simulink library "gmp_sil_core_pack_src"  (R2022b)
settings: Solver=VariableStepAuto  StartTime=0.0  StopTime=10.0  RelTol=1e-3
libraries: sm_lib x5, nesl_utility x4, fl_lib x3, peripheral_utilities x1, gmp_sil_core_pack x1
settings Model: Creator=javnson  LastModifiedBy=javnson

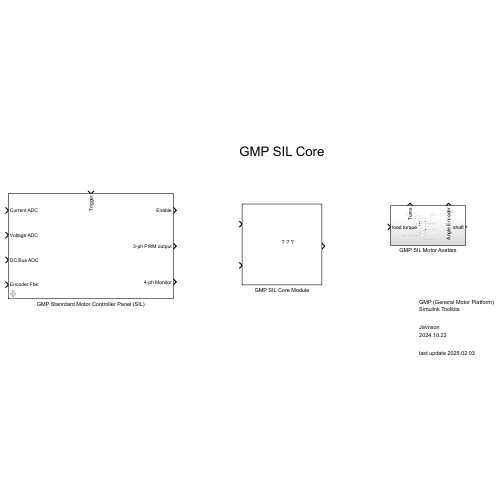
[thumbnail: Simulink's stored preview of the top-level diagram]
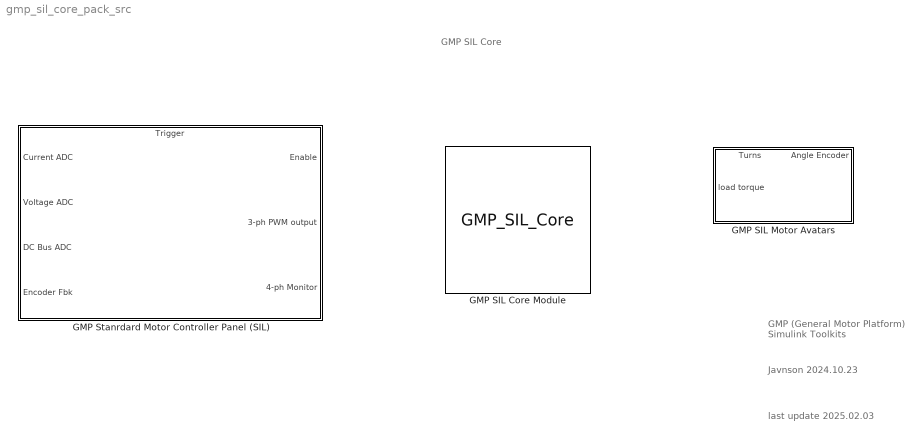
== system gmp_sil_core_pack_src ==
  note: last update 2025.02.03
  note: GMP SIL Core
  note: Javnson
      | 2024.10.23
  note: GMP (General Motor Platform)
      | Simulink Toolkits
  GMP SIL Core Module : S-Function  FunctionName=GMP_SIL_Core  Parameters=NumberUnpackedPorts, UnpackedDataTypes, UnpackedDataSizes, NumberPackedPorts, PackedDataTypes, PackedDataSizes, Alignment, HostAddr, TargetPort  SFunctionDeploymentMode=off  EnableBusSupport=off  mask(GMP CTL SIL Core){MaskPackedDataTypes={'double','double'}, MaskPackedDataSizes={[1],[1]}, MaskUnpackedDataTypes={'double'}, MaskUnpackedDataSizes={[1]}, MaskAlignment=1, MaskHostAddr='127.0.0.1', MaskMsgTxPort=12300, MaskMsgRxPort=12301, MaskCmdTxPort=12302, MaskCmdRxPort=12303}
      mask help:
      | This is the GMP (General Motor Platform) CTL (Control Template Library) SIL (Software In Loop) Core Model.
      | User should fill the following communication settings.
      mask init:
      | % MDL invoke parameters
      | % NumberUnpackedPorts, UnpackedDataTypes, UnpackedDataSizes, 
      | % NumberPackedPorts, PackedDataTypes, PackedDataSizes, 
      | % Alignment,
      | % HostAddr, TargetPort
      | 
      | % source: MaskUnpackedDataTypes, MaskUnpackedDataSizes
      | % source: MaskPackedDataTypes, MaskUnpackedDataSizes
      | % source: MaskAlignment
      | [NumberUnpackedPorts, UnpackedDataTypes, UnpackedDataSizes, ...
      |      NumberPackedPorts, PackedDataTypes, PackedDataSizes, ...
      |      Alignment] = mdl_gmp_simulink_core( ...
      |      MaskUnpackedDataTypes, MaskUnpackedDataSizes, ...
      |      MaskPackedDataTypes, MaskPackedDataSizes,...
      |      MaskAlignment);
      | 
      | % source: MaskHostAddr
      | % source: MaskMsgTxPort, MaskMsgRxPort
      | % source: MaskCmdTxPort, MaskCmdRxPort
      | [HostAddr, TargetPort] = mdl_gmp_simulink_connection(MaskHostAddr, ...
      | 	MaskMsgTxPort, MaskMsgRxPort, ... 
      | 	MaskCmdTxPort, MaskCmdRxPort);
      mask TypeOptions MaskAlignment: 1 | 2 | 4 | 8
      mask DialogControl ParameterGroupVar Prompt: Parameters:
      mask DialogControl Container5 Prompt: Message
      mask DialogControl Control3 Prompt: Data (sent) types (cell array):(pack)
      mask DialogControl Control7 Prompt: Data (send) port dimisions (cell array) (pack), disabled
      mask DialogControl Control5 Prompt: Data (received) types (cell array):(unpack)
      mask DialogControl Control6 Prompt: Data (received) port dimisions (cell array)(unpacked)
      mask DialogControl Control4 Prompt: Byte Alignment:
      mask DialogControl Container6 Prompt: Connection
      mask DialogControl Control8 Prompt: Target Host:
      mask DialogControl Control9 Prompt: MSG Transmit Port:
      mask DialogControl Control10 Prompt: MSG Receive Port:
      mask DialogControl Container7 Prompt: Command Ports
      mask DialogControl Control11 Prompt: CMD Transmit Port:
      mask DialogControl Control12 Prompt: CMD Receive Port:
      mask Display:
      | image(append(fileparts(which('gmp_simulink_utilities.slx')),'\icon\GMP_Core.png'));
      | 
      | 
      | disp('\n\n\n\n\n\n\n\nGMP SIL CORE Module');
  GMP SIL Motor Avatars : Subsystem
      settings: PortSchema="{\"entries\":[{\"content\":{\"sides\":[{\"content\":{\"connectorIds\":[\"In1\"]},\"type\":\"ConnectorPlacement.EquallySpacedRectSide\",\"uuid\":\"93fd98c8-22a3-43d8-9c64-5fedb21a7bba\"},{\"content\":{\"connectorIds\":[\"RConn1\"],\"side\":\"RIGHT\"},\"type\":\"ConnectorPlacement.EquallySpacedRectSide\",\"uuid\":\"d117f16d-9ccc-4fe6-b623-9fd4cd524b7a\"},{\"content\":{\"connectorIds\":[\"Out1\",\"Out2\"],\"side\":\"TOP\"},\"type\":\"ConnectorPlacement.EquallySpacedRectSide\",\"uuid\":\"de5de415-7a5e-456c-8b58-b022e0bdb100\"}]},\"type\":\"ConnectorPlacement.EquallySpacedConnector\",\"uuid\":\"15174bc1-c3ff-4fbf-b424-15a1ef65b97f\"}],\"packageUris\":[\"http://schema.mathworks.com/mf0/Connector/R2020b\"],\"version\":\"1.0\"}"
  GMP Stanrdard Motor Controller Panel (SIL) : Subsystem  mask(GMP SIL Core for single Motor Controller){}
      mask help: This is a General GMP SIL Motor Simulator.
      settings: PortSchema="{\"entries\":[{\"content\":{\"sides\":[{\"content\":{\"connectorIds\":[\"In1\",\"In2\",\"In3\",\"In4\"]},\"type\":\"ConnectorPlacement.EquallySpacedRectSide\",\"uuid\":\"92070e77-c4d8-4bd6-a20f-015d90d53703\"},{\"content\":{\"connectorIds\":[\"Out1\",\"Out2\",\"Out3\"],\"side\":\"RIGHT\"},\"type\":\"ConnectorPlacement.EquallySpacedRectSide\",\"uuid\":\"cd227558-01ea-4976-b12d-cc815f5c8239\"},{\"content\":{\"connectorIds\":[\"In5\"],\"side\":\"TOP\"},\"type\":\"ConnectorPlacement.EquallySpacedRectSide\",\"uuid\":\"6d86fdab-8964-4d81-bb99-d1a603f01c68\"}]},\"type\":\"ConnectorPlacement.EquallySpacedConnector\",\"uuid\":\"4dd76185-b108-46e1-8d6d-0c6e9edd0ad4\"}],\"packageUris\":[\"http://schema.mathworks.com/mf0/Connector/R2020b\"],\"version\":\"1.0\"}"

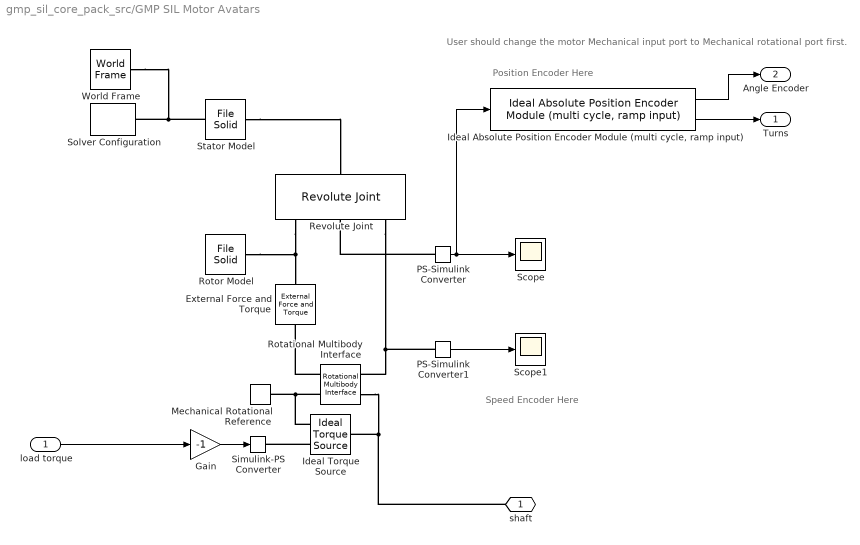
== system gmp_sil_core_pack_src/GMP SIL Motor Avatars ==
  note: User should change the motor Mechanical input port to Mechanical rotational port first.
  note: Speed Encoder Here
  note: Position Encoder Here
  load torque : Inport
  External Force and Torque : sm_lib/Forces and Torques/External Force and Torque  EnableForceX=off  EnableForceY=off  EnableForceZ=off  EnableForce=off  ForceResolutionFrame=AttachedFrame  EnableTorqueX=off  EnableTorqueY=off  EnableTorqueZ=on  EnableTorque=off  TorqueResolutionFrame=AttachedFrame
  Gain : Gain  Gain=-1
  "Ideal Absolute Position Encoder Module (multi cycle, ramp input)" : peripheral_utilities/Ideal Absolute Position Encoder Module (multi cycle, ramp input)  ENCODER_BIT=17
  Ideal Torque Source : fl_lib/Mechanical/Mechanical Sources/Ideal Torque Source
  Mechanical Rotational Reference : fl_lib/Mechanical/Rotational Elements/Mechanical Rotational Reference
  PS-Simulink Converter : nesl_utility/PS-Simulink Converter  PhysicalDomain=network_engine_domain  SubClassName=ps_output  LeftPortType=input  RightPortType=output  PseudoPeriodic=off  Frequencies=[]  VectorFormat=inherit  Unit=inherit  AffineConversion=off
  PS-Simulink Converter1 : nesl_utility/PS-Simulink Converter  PhysicalDomain=network_engine_domain  SubClassName=ps_output  LeftPortType=input  RightPortType=output  PseudoPeriodic=off  Frequencies=[]  VectorFormat=inherit  Unit=inherit  AffineConversion=off
  Revolute Joint : sm_lib/Joints/Revolute Joint  JointMode=Normal  CompositeWrenchDir=FollowerOnBase  CompositeWrenchFrame=BaseFrame  SenseConstraintForce=off  SenseConstraintTorque=off  SenseTotalForce=off  SenseTotalTorque=off  PositionTargetSpecify=off  PositionTargetPriority=High  PositionTargetValue=0  PositionTargetValueUnits=deg  VelocityTargetSpecify=off  VelocityTargetPriority=High  VelocityTargetValue=0  VelocityTargetValueUnits=deg/s  EquilibriumPosition=0  EquilibriumPositionUnits=deg  SpringStiffness=0  SpringStiffnessUnits=N*m/deg  DampingCoefficient=0  DampingCoefficientUnits=N*m/(deg/s)  LowerLimitSpecify=off  LowerLimitBound=-90  LowerLimitBoundUnits=deg  LowerLimitStiffness=1e4  LowerLimitStiffnessUnits=N*m/deg  LowerLimitDamping=10  LowerLimitDampingUnits=N*m/(deg/s)  LowerLimitTransitionRegionWidth=0.1  LowerLimitTransitionRegionWidthUnits=deg  UpperLimitSpecify=off  UpperLimitBound=90  UpperLimitBoundUnits=deg  UpperLimitStiffness=1e4  UpperLimitStiffnessUnits=N*m/deg  UpperLimitDamping=10  UpperLimitDampingUnits=N*m/(deg/s)  UpperLimitTransitionRegionWidth=0.1  UpperLimitTransitionRegionWidthUnits=deg  TorqueActuationMode=NoTorque  MotionActuationMode=ComputedMotion  SensePosition=on  SenseVelocity=on  SenseAcceleration=off  SenseTorqueForce=off  SenseLowerLimitTorqueForce=off  SenseUpperLimitTorqueForce=off
  Rotational Multibody Interface : fl_lib/Mechanical/Multibody Interfaces/Rotational Multibody Interface
  Rotor Model : sm_lib/Body Elements/File Solid  ExtGeomFileName=resources\rotor.STEP  UnitType=FromFile  ExtGeomFileUnits=m  StepReaderType=HEX  ExportConvexHullGeometry=off  InertiaType=CalculateFromGeometry  BasedOnType=Density  Density=1e-10  DensityUnits=kg/m^3  Mass=1  MassUnits=kg  CenterOfMass=[0 0 0]  CenterOfMassUnits=m  MomentsOfInertia=[1 1 1]  MomentsOfInertiaUnits=kg*m^2  ProductsOfInertia=[0 0 0]  ProductsOfInertiaUnits=kg*m^2  GraphicType=FromGeometry  MarkerShape=Sphere  MarkerSize=10  GraphicVisPropType=SimpleVisualProperties  GraphicDiffuseColor=[1.0 0.6 0.6]  GraphicOpacity=1  GraphicSpecularColor=[0.5 0.5 0.5 1.0]  GraphicAmbientColor=[0.15 0.15 0.15 1.0]  GraphicEmissiveColor=[0.0 0.0 0.0 1.0]  GraphicShininess=75  DoExposeReferenceFrame=off  SerializedFrames=<Frames><Frame><Id>Frame1</Id><Value><Name>F1</Name><Origin><Source>GeometricFeature</Source><FeatureName>planar surface 2</FeatureName></Origin><PrimaryAxis><DefinedDirection>+Z</DefinedDirection><Source>ReferenceFrame</Source><SourceDirection>+Z</SourceDirection><FeatureName></FeatureName></PrimaryAxis><SecondaryAxis><DefinedDirection>+X</DefinedDirection><Source>ReferenceFrame</Source><SourceDirection>+X</SourceDirection><FeatureName></FeatureName></SecondaryAxis></Value></Frame></Frames>
  Scope : Scope
  Scope1 : Scope
  Simulink-PS Converter : nesl_utility/Simulink-PS Converter  PhysicalDomain=network_engine_domain  SubClassName=ps_input  LeftPortType=input  RightPortType=output  PseudoPeriodic=off  Frequencies=[]  NoiseDistribution=none  NoiseParameters=[]  Unit=1  AffineConversion=off  FilteringAndDerivatives=provide  SimscapeFilterOrder=1  InputFilterTimeConstant=0.001  UdotUserProvided=0
  Solver Configuration : nesl_utility/Solver Configuration  PhysicalDomain=network_engine_domain  SubClassName=solver  LeftPortType=input  RightPortType=generic  Tones=[]  Harmonics=[]  SimulateNoise=off  Profile=off  UseLocalSampling=off  EnableSwitchedLinearOptims=on  FrequencyDomain=off  UseCCode=off  RelTol=0.001  AbsTol=0.001  MinStep=1e-09  ToWorkspace=off  RevertToSquareIcSolve=off  NumHomotopyIterations=100  PhasorMode=off  PhasorModeNumHarmonics=1  ConsistencySolver=NEWTON_XTOL_AFTER_FTOL  IndexReductionMethod=DerivativeReplacement  DoDC=off  ResidualTolerance=1e-09  ConsistencyTolSource=GLOBAL  ConsistencyAbsTol=0.001  ConsistencyRelTol=0.001  ConsistencyTolFactor=0.001  UseLocalSolver=off  LocalSolverChoice=NE_BACKWARD_EULER_ADVANCER  ResolveIndetEquations=on  FunctionEvalNumThread=1  LocalSolverSampleTime=1e-5  DoFixedCost=off  MaxNonlinIter=3  MaxModeIter=2  ComputeImpulses=off  ImpulseIterations=2  LinearAlgebra=auto  LinearAlgebraNumThread=0  EquationFormulation=NE_TIME_EF  DelaysMemoryBudget=1024  AutomaticFiltering=on  FilteringTimeConstant=0.001  PartitionStorageMethod=AS_NEEDED  PartitionMemoryBudget=1024  PartitionMethod=FAST
  Stator Model : sm_lib/Body Elements/File Solid  ExtGeomFileName=resources\stator.STEP  UnitType=FromFile  ExtGeomFileUnits=m  StepReaderType=HEX  ExportConvexHullGeometry=off  InertiaType=CalculateFromGeometry  BasedOnType=Density  Density=1000  DensityUnits=kg/m^3  Mass=1  MassUnits=kg  CenterOfMass=[0 0 0]  CenterOfMassUnits=m  MomentsOfInertia=[1 1 1]  MomentsOfInertiaUnits=kg*m^2  ProductsOfInertia=[0 0 0]  ProductsOfInertiaUnits=kg*m^2  GraphicType=FromGeometry  MarkerShape=Sphere  MarkerSize=10  GraphicVisPropType=SimpleVisualProperties  GraphicDiffuseColor=[0.8 0.8 0.8]  GraphicOpacity=1  GraphicSpecularColor=[0.5 0.5 0.5 1.0]  GraphicAmbientColor=[0.15 0.15 0.15 1.0]  GraphicEmissiveColor=[0.0 0.0 0.0 1.0]  GraphicShininess=75  DoExposeReferenceFrame=on  SerializedFrames=<Frames><Frame><Id>Frame1</Id><Value><Name>F1</Name><Origin><Source>GeometricFeature</Source><FeatureName>planar surface 14</FeatureName></Origin><PrimaryAxis><DefinedDirection>+Z</DefinedDirection><Source>ReferenceFrame</Source><SourceDirection>+Z</SourceDirection><FeatureName></FeatureName></PrimaryAxis><SecondaryAxis><DefinedDirection>+X</DefinedDirection><Source>ReferenceFrame</Source><SourceDirection>+X</SourceDirection><FeatureName></FeatureName></SecondaryAxis></Value></Frame></Frames>
  World Frame : sm_lib/Frames and Transforms/World Frame
  shaft : PMIOPort  Side=Right
  Turns : Outport
  Angle Encoder : Outport  Port=2
  wires:
  PS-Simulink Converter/1 -> "Ideal Absolute Position Encoder Module (multi cycle, ramp input)"/1, Scope/1
  PS-Simulink Converter1/1 -> Scope1/1
  Gain/1 -> Simulink-PS Converter/1
  load torque/1 -> Gain/1
  "Ideal Absolute Position Encoder Module (multi cycle, ramp input)"/1 -> Angle Encoder/1
  "Ideal Absolute Position Encoder Module (multi cycle, ramp input)"/2 -> Turns/1
  connections:
  World Frame/RConn1 -- Solver Configuration/RConn1 -- Stator Model/RConn1
  PS-Simulink Converter/LConn1 -- Revolute Joint/RConn2
  Revolute Joint/RConn1 -- Rotor Model/LConn1 -- External Force and Torque/RConn1
  Revolute Joint/RConn3 -- PS-Simulink Converter1/LConn1 -- Rotational Multibody Interface/RConn1
  Rotational Multibody Interface/RConn2 -- shaft/RConn1 -- Ideal Torque Source/LConn1
  Ideal Torque Source/RConn1 -- Simulink-PS Converter/RConn1
  Rotational Multibody Interface/LConn2 -- Ideal Torque Source/RConn2 -- Mechanical Rotational Reference/LConn1
  Rotational Multibody Interface/LConn1 -- External Force and Torque/LConn1
  Stator Model/LConn1 -- Revolute Joint/LConn1

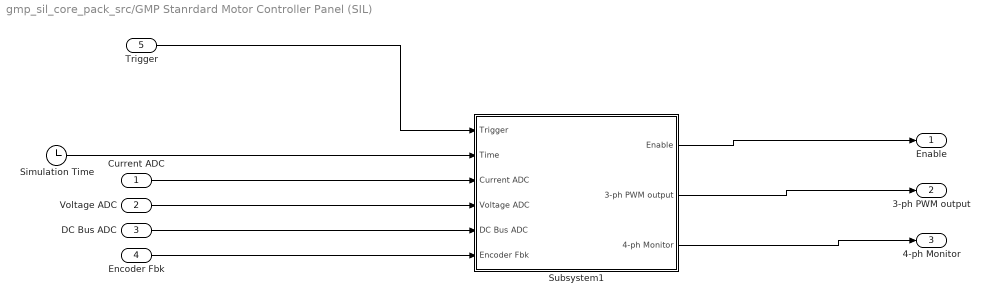
== system gmp_sil_core_pack_src/GMP Stanrdard Motor Controller Panel (SIL) ==
  Current ADC : Inport
  Voltage ADC : Inport  Port=2
  DC Bus ADC : Inport  Port=3
  Encoder Fbk : Inport  Port=4
  Trigger : Inport  Port=5
  Simulation Time : Clock
  Subsystem1 : Subsystem
  Enable : Outport
  3-ph PWM output : Outport  Port=2
  4-ph Monitor : Outport  Port=3
  wires:
  Trigger/1 -> Subsystem1/1(Trigger)
  Simulation Time/1 -> Subsystem1/2(Time)
  Current ADC/1 -> Subsystem1/3(Current ADC)
  Voltage ADC/1 -> Subsystem1/4(Voltage ADC)
  DC Bus ADC/1 -> Subsystem1/5(DC Bus ADC)
  Encoder Fbk/1 -> Subsystem1/6(Encoder Fbk)
  Subsystem1/1(Enable) -> Enable/1
  Subsystem1/2(3-ph PWM output) -> 3-ph PWM output/1
  Subsystem1/3(4-ph Monitor) -> 4-ph Monitor/1

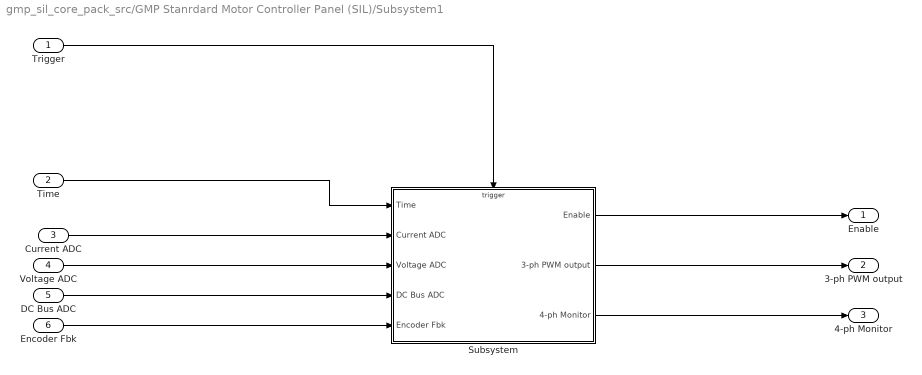
== system gmp_sil_core_pack_src/GMP Stanrdard Motor Controller Panel (SIL)/Subsystem1 ==
  Trigger : Inport
  Time : Inport  Port=2
  Current ADC : Inport  Port=3
  Voltage ADC : Inport  Port=4
  DC Bus ADC : Inport  Port=5
  Encoder Fbk : Inport  Port=6
  Subsystem : Subsystem
  Enable : Outport
  3-ph PWM output : Outport  Port=2
  4-ph Monitor : Outport  Port=3
  wires:
  DC Bus ADC/1 -> Subsystem/4(DC Bus ADC)
  Voltage ADC/1 -> Subsystem/3(Voltage ADC)
  Encoder Fbk/1 -> Subsystem/5(Encoder Fbk)
  Time/1 -> Subsystem/1(Time)
  Subsystem/3(4-ph Monitor) -> 4-ph Monitor/1
  Subsystem/1(Enable) -> Enable/1
  Subsystem/2(3-ph PWM output) -> 3-ph PWM output/1
  Current ADC/1 -> Subsystem/2(Current ADC)
  Trigger/1 -> Subsystem/Trigger

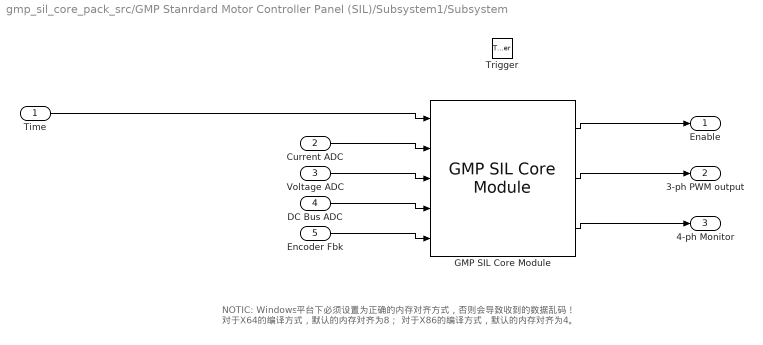
== system gmp_sil_core_pack_src/GMP Stanrdard Motor Controller Panel (SIL)/Subsystem1/Subsystem ==
  note: NOTIC:
      | Windows平台下必须设置为正确的内存对齐方式，否则会导致收到的数据乱码！
      | 对于X64的编译方式，默认的内存对齐为8；
      | 对于X86的编译方式，默认的内存对齐为4。
  Time : Inport
  Current ADC : Inport  Port=2
  Voltage ADC : Inport  Port=3
  DC Bus ADC : Inport  Port=4
  Encoder Fbk : Inport  Port=5
  Trigger : TriggerPort  VariantControl=(inherit)  PortDimensions=1
  GMP SIL Core Module : gmp_sil_core_pack/GMP SIL Core Module  MaskPackedDataTypes={'double','uint32','uint32','uint32','uint32'}  MaskPackedDataSizes={[1],[3],[3],[1],[1]}  MaskUnpackedDataTypes={'double', 'uint32','double'}  MaskUnpackedDataSizes={[1],[3],[4]}  MaskAlignment=1  MaskHostAddr='127.0.0.1'  MaskMsgTxPort=12300  MaskMsgRxPort=12301  MaskCmdTxPort=12302  MaskCmdRxPort=12303
  Enable : Outport
  3-ph PWM output : Outport  Port=2
  4-ph Monitor : Outport  Port=3
  wires:
  Encoder Fbk/1 -> GMP SIL Core Module/5
  Current ADC/1 -> GMP SIL Core Module/2
  Voltage ADC/1 -> GMP SIL Core Module/3
  DC Bus ADC/1 -> GMP SIL Core Module/4
  Time/1 -> GMP SIL Core Module/1
  GMP SIL Core Module/3 -> 4-ph Monitor/1
  GMP SIL Core Module/2 -> 3-ph PWM output/1
  GMP SIL Core Module/1 -> Enable/1
